simulink library "PID_Controller_Library"  (R2021b)
settings: Solver=VariableStepAuto  StartTime=0.0  StopTime=10.0  RelTol=1e-3
undefined symbols (not defined in the file): Ic, Kd, Ki, Kp
settings Model: Creator=amr_y  LastModifiedBy=amr_y

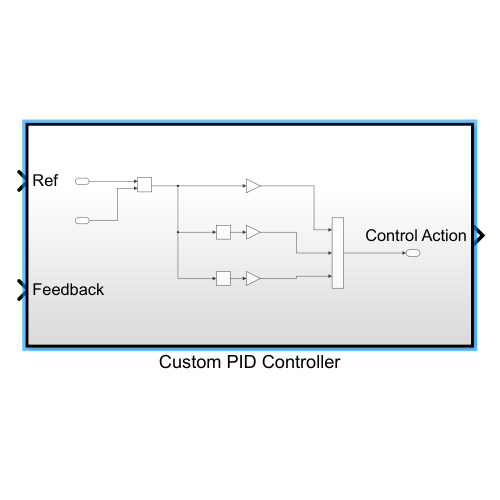
[thumbnail: Simulink's stored preview of the top-level diagram]
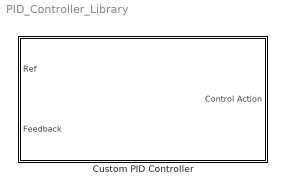
== system PID_Controller_Library ==
  Custom PID Controller : Subsystem  TreatAsAtomicUnit=on

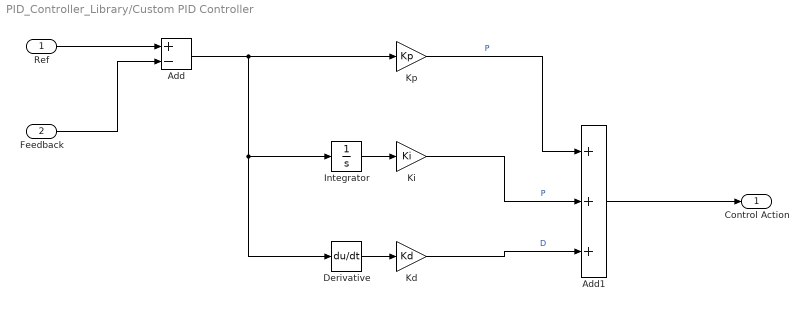
== system PID_Controller_Library/Custom PID Controller ==
  Ref : Inport
  Feedback : Inport  Port=2
  Add : Sum  Inputs=+-
  Add1 : Sum  Inputs=+++
  Derivative : Derivative
  Integrator : Integrator  InitialCondition=Ic
  Kd : Gain  Gain=Kd
  Ki : Gain  Gain=Ki
  Kp : Gain  Gain=Kp
  Control Action : Outport
  wires:
  Add/1 -> Kp/1, Derivative/1, Integrator/1
  Ref/1 -> Add/1
  Kp/1 -> Add1/1  "P"
  Feedback/1 -> Add/2
  Kd/1 -> Add1/3  "D"
  Add1/1 -> Control Action/1
  Integrator/1 -> Ki/1
  Ki/1 -> Add1/2  "P"
  Derivative/1 -> Kd/1
